simulink library "pv_performance_module"  (R2025b)
settings: Solver=VariableStepAuto  StartTime=0.0  StopTime=10.0  RelTol=1e-3
settings Model: Creator=ciepm  LastModifiedBy=dmlevine

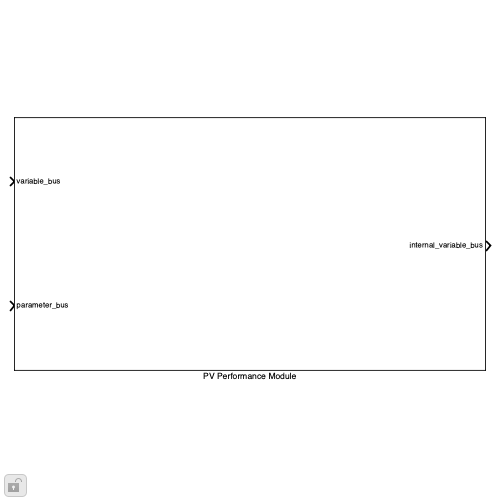
[thumbnail: Simulink's stored preview of the top-level diagram]
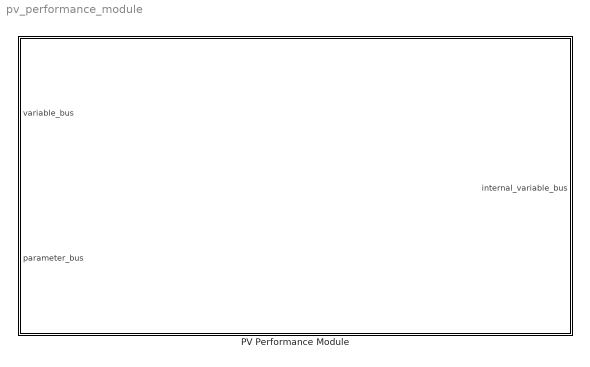
== system pv_performance_module ==
  PV Performance Module : Subsystem

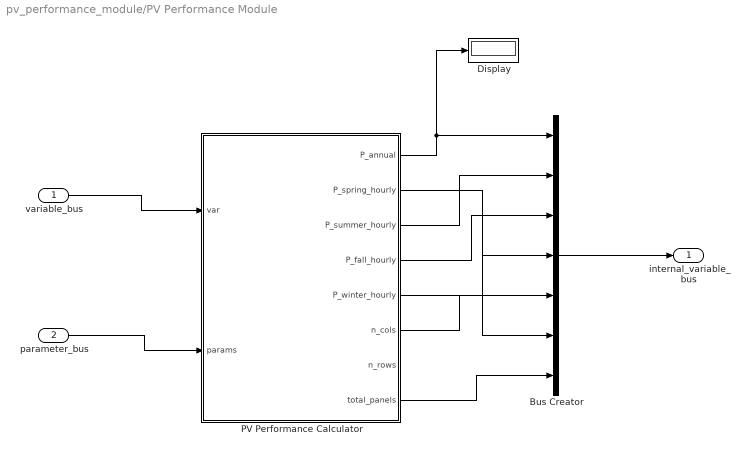
== system pv_performance_module/PV Performance Module ==
  variable_bus : Inport
  parameter_bus : Inport  Port=2
  Bus Creator : BusCreator  Inputs=7
  Display : Display
  PV Performance Calculator : MATLAB Function  TreatAsAtomicUnit=on
  internal_variable_bus : Outport
  wires:
  PV Performance Calculator/1(P_annual) -> Bus Creator/1, Display/1
  variable_bus/1 -> PV Performance Calculator/1(var)
  Bus Creator/1 -> internal_variable_bus/1
  parameter_bus/1 -> PV Performance Calculator/2(params)
  PV Performance Calculator/2(P_spring_hourly) -> Bus Creator/6
  PV Performance Calculator/3(P_summer_hourly) -> Bus Creator/2
  PV Performance Calculator/4(P_fall_hourly) -> Bus Creator/3
  PV Performance Calculator/5(P_winter_hourly) -> Bus Creator/4
  PV Performance Calculator/6(n_cols) -> Bus Creator/5
  PV Performance Calculator/8(total_panels) -> Bus Creator/7

== matlab function pv_performance_module/PV Performance Module/PV Performance Calculator ==
  data: var input; P_annual output; params input; P_spring_hourly output; P_summer_hourly output; P_fall_hourly output; P_winter_hourly output; n_cols output; n_rows output; total_panels output
function [P_annual, P_spring_hourly, P_summer_hourly, P_fall_hourly, P_winter_hourly, n_cols, n_rows, total_panels] = pv_model1(var, params)
    
    % This Simulink block is just a passthrough, all the actual math is tracked on GitHub inside pv_power.m
    
    [P_annual, P_spring_hourly, P_summer_hourly, P_fall_hourly, P_winter_hourly, n_cols, n_rows, total_panels] = pv_power(var, params);

end
